simulink model "sprawko3z3a"  (R2019b)
settings: Solver=VariableStepAuto  StartTime=0.0  StopTime=10.0  RelTol=1e-3
values from neighbouring files (symbols this model uses):
  a0 = 1    [anal_c_d.m]    (also in symulacyjne3B.m)
  a1 = 1    [anal_c_d.m]    (also in symulacyjne3B.m)
  b = 2    [anal_c_d.m]    (also in symulacyjne3B.m)
settings Model: Creator=margr  LastModifiedBy=margr

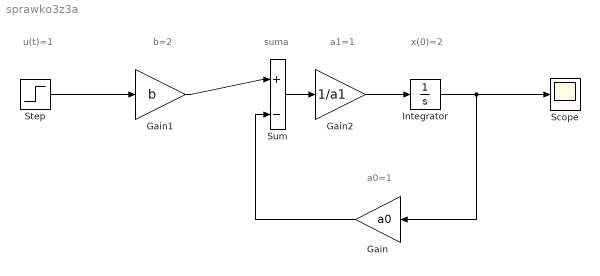
== system sprawko3z3a ==
  note: suma
  note: b=2
  note: a1=1
  note: a0=1
  note: x(0)=2
  note: u(t)=1
  Gain : Gain  Gain=a0
  Gain1 : Gain  Gain=b
  Gain2 : Gain  Gain=1/a1
  Integrator : Integrator  InitialCondition=2
  Scope : Scope
  Step : Step  Time=0  SampleTime=0
  Sum : Sum  Inputs=|+-
  wires:
  Integrator/1 -> Gain/1, Scope/1
  Step/1 -> Gain1/1
  Gain1/1 -> Sum/1
  Sum/1 -> Gain2/1
  Gain/1 -> Sum/2
  Gain2/1 -> Integrator/1
